simulink model "MBDMotorSystemUpd1MaxIaLmt"  (R2023a)
settings: Solver=VariableStepAuto  StartTime=0.0  StopTime=0.5  RelTol=1e-3
undefined symbols (not defined in the file or in its folder): CntFdqDcpMap, CntLdqDMap, CntTrqReqMap, DiscIntNeverNeededParam, Izc, Izr, MdlFluxMap, MdlTrqMap, Pos0
libraries: simulink x30, simulink_extras x6
(part 2 of 4)

== system MBDMotorSystemUpd1MaxIaLmt/PM Controller/IPM Trq To Id-Iq Request ==
  Vdc : Inport
  TrqIn : Inport  Port=2
  w : Inport  Port=3
  Time : Inport  Port=4
  Trigger : TriggerPort  VariantControl=Variant  PortDimensions=1
  Abs : Abs  SaturateOnIntegerOverflow=off
  Display : Display
  Gain : Gain  Gain=120/nP
  Gain1 : Gain  Gain=-1
  Id Map : Lookup_n-D  NumberOfTableDimensions=3  BreakpointsForDimension1=TrqIdx  BreakpointsForDimension2=NsIdx  BreakpointsForDimension3=VdcIdx  Table=IdMap  InternalRulePriority=Speed  RndMeth=Simplest
      settings: InputPortMap=u0,u1,u2
  Iq Map : Lookup_n-D  NumberOfTableDimensions=3  BreakpointsForDimension1=TrqIdx  BreakpointsForDimension2=NsIdx  BreakpointsForDimension3=VdcIdx  Table=IqMap  InternalRulePriority=Speed  RndMeth=Simplest
      settings: InputPortMap=u0,u1,u2
  Mux : Mux  Inputs=2
  Product : Product
  Product1 : Product
  Saturation Dynamic : simulink/Discontinuities/Saturation Dynamic  OutMin=[]  OutMax=[]  OutDataTypeStr=Inherit: Same as second input  OutDataType=fixdt(1, 16)  OutScaling=2^-10  DoSatur=off
  Sign : Signum
  Sign1 : Signum
  Torque Rate Limitter : Subsystem  mask{DltLmt=DltTrqLmt}
      mask prompts: DltLmt "変化率制限 [unit/s]"
  Trq Limt Map : Lookup_n-D  BreakpointsForDimension1=NsIdx  BreakpointsForDimension2=VdcIdx  BreakpointsForDimension3=VdcIdx  Table=MapLimitTrq  InternalRulePriority=Speed  RndMeth=Simplest
      settings: InputPortMap=u0,u1
  WtoF : Gain  Gain=1/(2*pi)
  TrqReq : Outport
  IdqReq : Outport  Port=2
  wires:
  Mux/1 -> IdqReq/1
  Id Map/1 -> Mux/1
  w/1 -> WtoF/1
  TrqIn/1 -> Torque Rate Limitter/1(In)
  Saturation Dynamic/1 -> Product/1, Id Map/1, Iq Map/1
  Gain1/1 -> Saturation Dynamic/3
  Vdc/1 -> [Vdc]
  [Vdc] -> Trq Limt Map/2
  [Nrpm] -> Iq Map/2, Id Map/2
  [Nrpm] -> Trq Limt Map/1
  Gain/1 -> Display/1, [Nrpm]
  [Vdc] -> Id Map/3, Iq Map/3
  Trq Limt Map/1 -> Gain1/1, Saturation Dynamic/1
  Torque Rate Limitter/1(Rate Limited) -> Abs/1, Sign1/1, Sign/1
  Time/1 -> Torque Rate Limitter/2(Time)
  Abs/1 -> Saturation Dynamic/2
  Product/1 -> TrqReq/1
  Sign/1 -> Product/2
  Product1/1 -> Mux/2
  Iq Map/1 -> Product1/1
  Sign1/1 -> Product1/2
  WtoF/1 -> Gain/1

== system MBDMotorSystemUpd1MaxIaLmt/PM Controller/LPF ==
  In : Inport  SampleTime=Ts
  Init : Inport  Port=2  SampleTime=Ts
  Constant : Constant  Value=Ts
  Constant1 : Constant  Value=tau
  Delay : Delay  DelayLength=1  InitialConditionSource=Input port
      settings: InputPortMap=u0,p4
  Divide1 : Product  Inputs=*/
  Divide3 : Product  Inputs=*/
  Product : Product
  Product1 : Product
  Sum1 : Sum
  Sum2 : Sum
  Sum3 : Sum  Inputs=-+
  Out : Outport
  wires:
  Constant1/1 -> Divide1/1, Sum1/2
  Constant/1 -> Sum1/1, Divide3/1
  Sum1/1 -> Divide1/2, Divide3/2
  Divide3/1 -> [kX]
  Divide1/1 -> [kY]
  In/1 -> Product/1
  [kX] -> Product/2
  Product/1 -> Sum3/1, Sum2/1
  Sum2/1 -> Out/1, Product1/1
  [kY] -> Product1/2
  Product1/1 -> Delay/1
  Delay/1 -> Sum2/2
  Init/1 -> Sum3/2
  Sum3/1 -> Delay/2

== system MBDMotorSystemUpd1MaxIaLmt/PM Controller/Modulator ==
  Vdc : Inport
  Vdq* : Inport  Port=2
  Th [deg.] : Inport  Port=3
  w : Inport  Port=4
  Tc : Inport  Port=5
  Trigger : TriggerPort  TriggerType=falling  VariantControl=Variant
  DQ to UVW : Subsystem
  Divide : Product  Inputs=*/
  Gain : Gain  Gain=0.5
  Gain2 : Gain  Gain=1.5
  IsOvrMod : Constant  Value=0
  Over Modulation : Subsystem
  Product : Product
  Saturation : Saturate  UpperLimit=inf  LowerLimit=1  LinearizeAsGain=off
  Sum : Sum  Inputs=|++
  Sum7 : Sum  Inputs=|+-
  TypePWM : Constant  Value=0
  Vz Correction : Subsystem
  Muvw : Outport
  Vuvw* : Outport  Port=2
  wires:
  Gain/1 -> Vz Correction/3(MaxVa), Divide/2
  Sum/1 -> Divide/1
  Vz Correction/1(Vz) -> Sum/2
  DQ to UVW/1(UVW) -> Sum/1, Vuvw*/1, Vz Correction/2(VaReq)
  Vdq*/1 -> DQ to UVW/1(dq)
  Vdc/1 -> Saturation/1
  Saturation/1 -> Gain/1
  Product/1 -> Gain2/1
  Th [deg.]/1 -> Sum7/1
  Sum7/1 -> DQ to UVW/2(Th)
  w/1 -> Product/1
  Tc/1 -> Product/2
  Gain2/1 -> Sum7/2
  Divide/1 -> Over Modulation/3(Mr)
  IsOvrMod/1 -> Over Modulation/1(Is OvrMod)
  TypePWM/1 -> Over Modulation/2(PWM Mode), Vz Correction/1(PWM Mode)
  Over Modulation/1(Mr*) -> Muvw/1

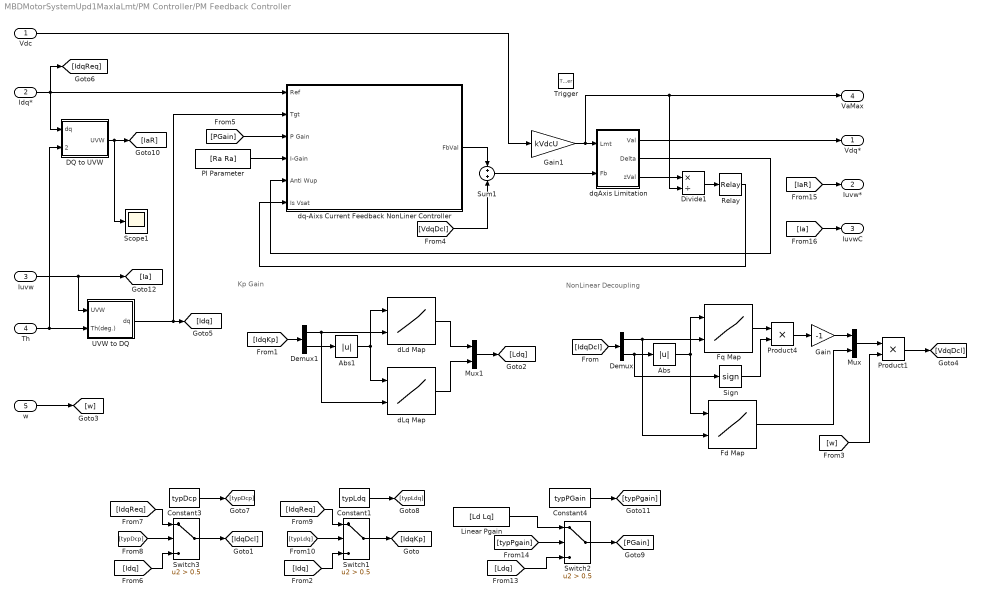
== system MBDMotorSystemUpd1MaxIaLmt/PM Controller/PM Feedback Controller ==
  note: Kp Gain
  note: NonLinear Decoupling
  Vdc : Inport
  Idq* : Inport  Port=2
  Iuvw : Inport  Port=3
  Th : Inport  Port=4
  w : Inport  Port=5
  Trigger : TriggerPort  TriggerType=falling  VariantControl=Variant  PortDimensions=1
  Abs : Abs  SaturateOnIntegerOverflow=off
  Abs1 : Abs  SaturateOnIntegerOverflow=off
  Constant1 : Constant  Value=typLdq
  Constant3 : Constant  Value=typDcp
  Constant4 : Constant  Value=typPGain
  DQ to UVW : Subsystem
  Demux : Demux  Outputs=2
  Demux1 : Demux  Outputs=2
  Divide1 : Product  Inputs=*/
  Fd Map : Lookup_n-D  BreakpointsForDimension1=axIqY  BreakpointsForDimension2=axIdX  Table=mIdqToFd  InternalRulePriority=Speed  RndMeth=Simplest
      settings: InputPortMap=u0,u1
  Fq Map : Lookup_n-D  BreakpointsForDimension1=axIqY  BreakpointsForDimension2=axIdX  Table=mIdqToFq  InternalRulePriority=Speed  RndMeth=Simplest
      settings: InputPortMap=u0,u1
  Gain : Gain  Gain=-1
  Gain1 : Gain  Gain=kVdcU
  Linear Pgain : Constant  Value=[Ld Lq]
  Mux : Mux  Inputs=2
  Mux1 : Mux  Inputs=2
  PI Parameter : Constant  Value=[Ra Ra]
  Product1 : Product
  Product4 : Product
  Relay : Relay  OnSwitchValue=0.98  OffSwitchValue=0.95
  Scope1 : Scope
  Sign : Signum
  Sum1 : Sum  Inputs=+|+
  Switch1 : Switch  Criteria=u2 > Threshold  Threshold=0.5  SaturateOnIntegerOverflow=off  InputSameDT=off
  Switch2 : Switch  Criteria=u2 > Threshold  Threshold=0.5  SaturateOnIntegerOverflow=off  InputSameDT=off
  Switch3 : Switch  Criteria=u2 > Threshold  Threshold=0.5  SaturateOnIntegerOverflow=off  InputSameDT=off
  UVW to DQ : Subsystem
  dLd Map : Lookup_n-D  BreakpointsForDimension1=axIdXdL  BreakpointsForDimension2=axIqYdL  Table=mIdqToLd  InternalRulePriority=Speed  RndMeth=Simplest
      settings: InputPortMap=u0,u1
  dLq Map : Lookup_n-D  BreakpointsForDimension1=axIdXdL  BreakpointsForDimension2=axIqYdL  Table=mIdqToLq  InternalRulePriority=Speed  RndMeth=Simplest
      settings: InputPortMap=u0,u1
  dq-Aixs Current Feedback NonLiner Controller : Subsystem  mask{KcDt=KcDt, KcQt=KcQt, KcDw=KcDw, KcQw=KcQw}
      mask prompts: KcDt "Id Cut off Gain [rad./s]"; KcQt "Iq Cut off Gain [rad./s]"; KcDw "Id Cut off Gain [rad./s]"; KcQw "Iq Cut off Gain [rad./s]"
      mask init:
      | KcT=[KcDt KcQt];
      |     KcW=[KcDw KcQw];
      mask DialogControl Container1 Prompt: Current Feedback Gain
      mask DialogControl Container2 Prompt: MTPA
      mask DialogControl Container3 Prompt: Field Weakening
      mask Display:
      | disp(['dq-Axis Current Feedback\nControler\n\n', ...
      |       sprintf('MTPA - d:%g / q:%g [rad./s]\n',KcDt,KcQt), ...
      |       sprintf('FdWk - d:%g / q:%g [rad./s]\n',KcDw,KcQw), ...
      |       '']);
  dqAxis Limitation : Subsystem
  Vdq* : Outport
  Iuvw* : Outport  Port=2
  IuvwC : Outport  Port=3
  VaMax : Outport  Port=4
  wires:
  DQ to UVW/1(UVW) -> [IaR], Scope1/1
  Th/1 -> DQ to UVW/2(Th. [deg.]), UVW to DQ/2(Th(deg.))
  Iuvw/1 -> [Ia], UVW to DQ/1(UVW)
  Gain1/1 -> Divide1/2, VaMax/1, dqAxis Limitation/1(Lmt)
  Sum1/1 -> dqAxis Limitation/2(Fb)
  dqAxis Limitation/1(Val) -> Vdq*/1
  Idq*/1 -> [IdqReq], DQ to UVW/1(dq), dq-Aixs Current Feedback NonLiner Controller/1(Ref)
  Vdc/1 -> Gain1/1
  dqAxis Limitation/2(Delta) -> dq-Aixs Current Feedback NonLiner Controller/5(Anti Wup)
  UVW to DQ/1(dq) -> [Idq], dq-Aixs Current Feedback NonLiner Controller/2(Tgt)
  Gain/1 -> Mux/1
  Fd Map/1 -> Mux/2
  dLd Map/1 -> Mux1/1
  dLq Map/1 -> Mux1/2
  [IdqDcl] -> Demux/1
  [IdqKp] -> Demux1/1
  Mux1/1 -> [Ldq]
  w/1 -> [w]
  [w] -> Product1/2
  [VdqDcl] -> Sum1/2
  Switch3/1 -> [IdqDcl]
  [Idq] -> Switch3/3
  [IdqReq] -> Switch3/1
  [typDcp] -> Switch3/2
  Constant3/1 -> [typDcp]
  [typLdq] -> Switch1/2
  [Idq] -> Switch1/3
  [IdqReq] -> Switch1/1
  Switch1/1 -> [IdqKp]
  Constant1/1 -> [typLdq]
  [Ldq] -> Switch2/3
  Linear Pgain/1 -> Switch2/1
  Switch2/1 -> [PGain]
  Constant4/1 -> [typPgain]
  [typPgain] -> Switch2/2
  [PGain] -> dq-Aixs Current Feedback NonLiner Controller/3(P Gain)
  PI Parameter/1 -> dq-Aixs Current Feedback NonLiner Controller/4(I-Gain)
  Divide1/1 -> Relay/1
  dqAxis Limitation/3(zVal) -> Divide1/1
  Relay/1 -> dq-Aixs Current Feedback NonLiner Controller/6(Is Vsat)
  Demux/1 -> Fd Map/2, Fq Map/2
  Demux/2 -> Sign/1, Abs/1
  Product4/1 -> Gain/1
  Fq Map/1 -> Product4/1
  Sign/1 -> Product4/2
  Abs/1 -> Fd Map/1, Fq Map/1
  Demux1/2 -> Abs1/1
  Abs1/1 -> dLq Map/1, dLd Map/1
  Demux1/1 -> dLd Map/2, dLq Map/2
  Product1/1 -> [VdqDcl]
  Mux/1 -> Product1/1
  dq-Aixs Current Feedback NonLiner Controller/1(FbVal) -> Sum1/1
  [IaR] -> Iuvw*/1
  [Ia] -> IuvwC/1

== system MBDMotorSystemUpd1MaxIaLmt/PM Controller/PWM Timer ==
  Req : Inport  PortDimensions=3
  Fc : Inport  Port=2
  Iuvw : Inport  Port=3
  Base Modulator : Subsystem  mask{lTypTrigger=1: 山}
      mask prompts: lTypTrigger "更新トリガ"
      mask TypeOptions lTypTrigger: sampler/lTypTrigger
  Dead  Time : Constant  Value=[Td; -Td]
  DeadTime Correction : Subsystem  mask{IsDeadTimeCorrection=on, vThr=vThr}
      mask prompts: IsDeadTimeCorrection "DeadTime補償有効"; vThr "補償方向電流閾値"
      mask init:
      | if strcmp(get_param(gcbh,'IsDeadTimeCorrection'),'on')
      |     kCrctTd=1;
      | else
      |     kCrctTd=0;
      | end
  Demux : Demux  Outputs=2
  Demux1 : Demux  Outputs=3
  Demux2 : Demux  Outputs=3
  Gain : Gain  Gain=2
  Mux{1..4} (4 alike) : Mux  Inputs=2
  Mux5 : Mux  Inputs=3
  PWM Sampler : Subsystem  TreatAsAtomicUnit=on
  PWM Status : Scope  NumInputPorts=4
  Product1 : Product
  Relational Operator : RelationalOperator  OutDataTypeStr=boolean  RndMeth=Simplest  InputSameDT=off
  Relational Operator1 : RelationalOperator  Operator=<=  OutDataTypeStr=boolean  RndMeth=Simplest  InputSameDT=off
  Signal Offset : Subsystem
  Sum1 : Sum  Inputs=|++
  Sum2 : Sum  Inputs=|++
  Trg : Outport
  PWM : Outport  Port=2
  Tc : Outport  Port=3
  wires:
  [Trg] -> PWM Status/3
  [ModV] -> PWM Status/2
  Mux4/1 -> [ModV]
  [CrcTd] -> PWM Status/4
  Sum2/1 -> Mux4/2, Relational Operator/1, Relational Operator1/1
  PWM Sampler/1(s) -> Sum2/1
  DeadTime Correction/1(Tdc) -> Sum2/2, [CrcTd]
  Iuvw/1 -> DeadTime Correction/2(Iuvw)
  Base Modulator/1("Trigger ") -> [Trg], PWM Sampler/Trigger, Trg/1
  Sum1/1 -> Mux4/1, Demux/1
  Product1/1 -> Sum1/2, DeadTime Correction/1(Tdcs)
  Base Modulator/2(Carrier) -> Sum1/1
  Fc/1 -> Product1/1, Base Modulator/1(Fc)
  Gain/1 -> Product1/2
  Dead  Time/1 -> Gain/1
  Mux5/1 -> Signal Offset/1(puvw), PWM/1
  Req/1 -> PWM Sampler/1(v)
  Mux3/1 -> Mux5/3  "Pw"
  Mux2/1 -> Mux5/2  "Pv"
  Mux1/1 -> Mux5/1  "Pu"
  Signal Offset/1(Pwm SigOuts) -> PWM Status/1
  Demux2/3 -> Mux3/2
  Demux2/2 -> Mux2/2
  Demux2/1 -> Mux1/2
  Demux1/3 -> Mux3/1
  Demux1/2 -> Mux2/1
  Demux1/1 -> Mux1/1
  Relational Operator1/1 -> Demux2/1
  Demux/2 -> Relational Operator1/2
  Demux/1 -> Relational Operator/2
  Relational Operator/1 -> Demux1/1
  Base Modulator/3(Tc) -> Tc/1

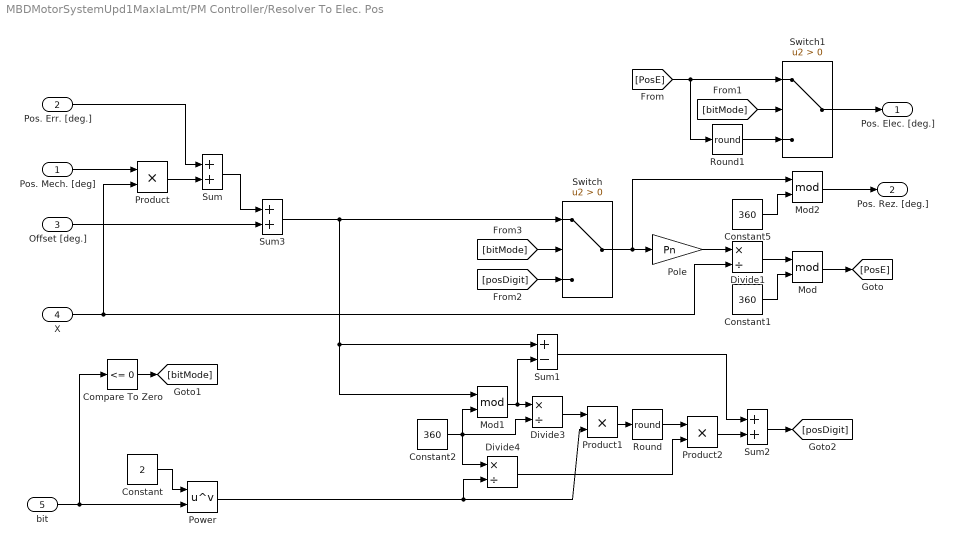
== system MBDMotorSystemUpd1MaxIaLmt/PM Controller/Resolver To Elec. Pos ==
  Pos. Mech. [deg] : Inport
  Pos. Err. [deg.] : Inport  Port=2
  Offset [deg.] : Inport  Port=3
  X : Inport  Port=4
  bit : Inport  Port=5
  Compare To Zero : simulink/Logic and Bit Operations/Compare To Zero  relop=<=  OutDataTypeStr=uint8
  Constant : Constant  Value=2
  Constant1 : Constant  Value=360
  Constant2 : Constant  Value=360
  Constant5 : Constant  Value=360
  Divide1 : Product  Inputs=*/
  Divide3 : Product  Inputs=*/
  Divide4 : Product  Inputs=*/
  Mod : Math  Operator=mod
  Mod1 : Math  Operator=mod
  Mod2 : Math  Operator=mod
  Pole : Gain  Gain=Pn
  Power : Math  Operator=pow
  Product : Product
  Product1 : Product
  Product2 : Product
  Round : Rounding  Operator=round
  Round1 : Rounding  Operator=round
  Sum : Sum
  Sum1 : Sum  Inputs=+-
  Sum2 : Sum
  Sum3 : Sum
  Switch : Switch  Criteria=u2 > Threshold  SaturateOnIntegerOverflow=off  InputSameDT=off
  Switch1 : Switch  Criteria=u2 > Threshold  SaturateOnIntegerOverflow=off  InputSameDT=off
  Pos. Elec. [deg.] : Outport
  Pos. Rez. [deg.] : Outport  Port=2
  wires:
  Pos. Mech. [deg]/1 -> Product/1
  Power/1 -> Divide4/2, Product1/2
  X/1 -> Product/2, Divide1/2
  bit/1 -> Power/2, Compare To Zero/1
  Constant/1 -> Power/1
  Constant1/1 -> Mod/2
  Product/1 -> Sum/2
  Switch/1 -> Mod2/1, Pole/1
  Pole/1 -> Divide1/1
  Divide1/1 -> Mod/1
  Round1/1 -> Switch1/3
  Switch1/1 -> Pos. Elec. [deg.]/1
  Mod/1 -> [PosE]
  [PosE] -> Round1/1, Switch1/1
  [bitMode] -> Switch1/2
  [posDigit] -> Switch/3
  Constant2/1 -> Divide4/1, Divide3/2, Mod1/2
  Compare To Zero/1 -> [bitMode]
  [bitMode] -> Switch/2
  Mod2/1 -> Pos. Rez. [deg.]/1
  Constant5/1 -> Mod2/2
  Pos. Err. [deg.]/1 -> Sum/1
  Mod1/1 -> Sum1/2, Divide3/1
  Divide3/1 -> Product1/1
  Product1/1 -> Round/1
  Round/1 -> Product2/1
  Divide4/1 -> Product2/2
  Product2/1 -> Sum2/2
  Sum1/1 -> Sum2/1
  Sum2/1 -> [posDigit]
  Sum3/1 -> Mod1/1, Sum1/1, Switch/1
  Offset [deg.]/1 -> Sum3/2
  Sum/1 -> Sum3/1

== system MBDMotorSystemUpd1MaxIaLmt/PM Controller/Resolver Settings ==
  Pos. Mech. [deg.] : Inport
  Bit : Constant  Value=10
  Bus Creator : BusCreator  Inputs=3
  Constant : Constant  Value=0
  Constant1 : Constant  Value=0
  Constant4 : Constant  Value=360
  Err Stt : Constant
  Fail : Step  Time=1.2  SampleTime=0
  Fail Speed a [rpm] : Constant  Value=0
  Fail Speed b [rpm] : Constant  Value=30
  Fail Stt : Constant
  Manual Switch{,1..3} (4 alike) : ManualSwitch
  Mod1 : Math  Operator=mod
  Offset : Constant  Value=0
  Product : Product
  Resolver Error : Subsystem
  Resolver Fail : Subsystem
  X : Constant  Value=50
  Pos. Mech. [deg] : Outport
  Err. [deg.] : Outport  Port=2
  Ia Sensor Parm. : Outport  Port=3
  wires:
  Bus Creator/1 -> Ia Sensor Parm./1
  Pos. Mech. [deg.]/1 -> Product/2, Resolver Fail/1(Pos. Mech. [deg.])
  Resolver Error/1(Err. [deg.]) -> Err. [deg.]/1
  Offset/1 -> Bus Creator/1  "Offset"
  X/1 -> [x], Bus Creator/2  "X"
  Bit/1 -> Bus Creator/3  "Bit"
  Resolver Fail/1(Pos. Mech. [deg]) -> Pos. Mech. [deg]/1
  Fail Speed a [rpm]/1 -> Manual Switch/1
  Fail Speed b [rpm]/1 -> Manual Switch/2
  Manual Switch/1 -> Resolver Fail/2(Fail Speed [rpm])
  Fail Stt/1 -> Manual Switch1/1
  Fail/1 -> Manual Switch1/2
  Manual Switch2/1 -> Resolver Fail/3(Fail)
  Constant/1 -> Manual Switch2/1
  Manual Switch1/1 -> Manual Switch2/2
  Constant1/1 -> Manual Switch3/1
  Err Stt/1 -> Manual Switch3/2
  Manual Switch3/1 -> Resolver Error/2(Fail)
  [x] -> Product/1
  Constant4/1 -> Mod1/2
  Product/1 -> Mod1/1
  Mod1/1 -> Resolver Error/1(Pos Rez. [deg.])

== system MBDMotorSystemUpd1MaxIaLmt/PM Controller/TrgPos ==
  Pos (deg.) : Inport
  Trigger : TriggerPort  TriggerType=falling  VariantControl=Variant
  Pos (Smpled) : Outport
  wires:
  Pos (deg.)/1 -> Pos (Smpled)/1

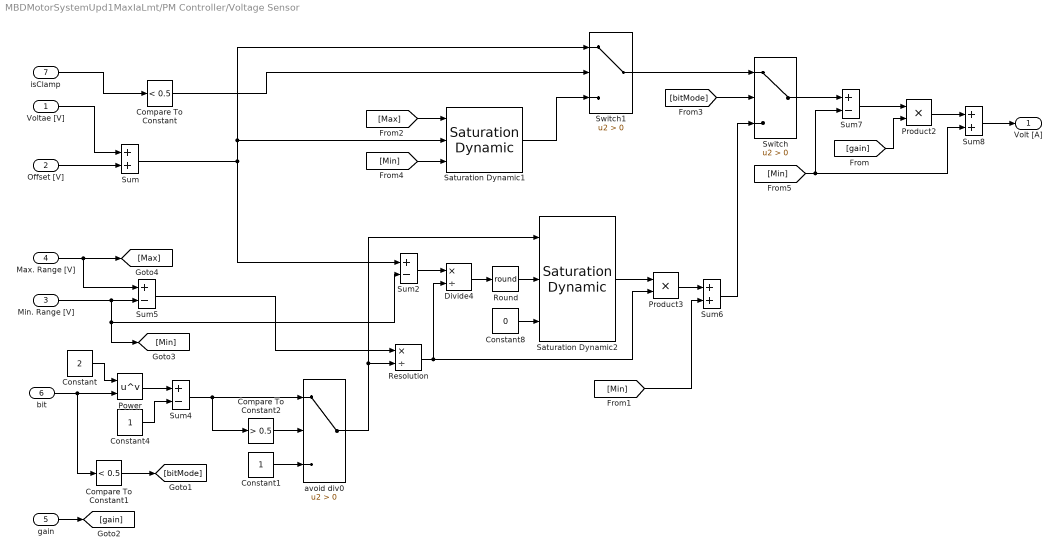
== system MBDMotorSystemUpd1MaxIaLmt/PM Controller/Voltage Sensor ==
  Voltae [V] : Inport
  Offset [V] : Inport  Port=2
  Min. Range [V] : Inport  Port=3
  Max. Range [V] : Inport  Port=4
  gain : Inport  Port=5
  bit : Inport  Port=6
  isClamp : Inport  Port=7
  Compare To Constant : simulink/Logic and Bit Operations/Compare To Constant  relop=<  const=0.5  OutDataTypeStr=boolean
  Compare To Constant1 : simulink/Logic and Bit Operations/Compare To Constant  relop=<  const=0.5  OutDataTypeStr=boolean
  Compare To Constant2 : simulink/Logic and Bit Operations/Compare To Constant  relop=>  const=0.5  OutDataTypeStr=boolean
  Constant : Constant  Value=2
  Constant1 : Constant
  Constant4 : Constant
  Constant8 : Constant  Value=0
  Divide4 : Product  Inputs=*/
  Power : Math  Operator=pow
  Product2 : Product
  Product3 : Product
  Resolution : Product  Inputs=*/
  Round : Rounding  Operator=round
  Saturation Dynamic1 : simulink/Discontinuities/Saturation Dynamic  OutMin=[]  OutMax=[]  OutDataTypeStr=Inherit: Same as second input  OutDataType=fixdt(1, 16)  OutScaling=2^-10  DoSatur=off
  Saturation Dynamic2 : simulink/Discontinuities/Saturation Dynamic  OutMin=[]  OutMax=[]  OutDataTypeStr=Inherit: Same as second input  OutDataType=fixdt(1, 16)  OutScaling=2^-10  DoSatur=off
  Sum : Sum
  Sum{2,4..5,7} (4 alike) : Sum  Inputs=+-
  Sum6 : Sum
  Sum8 : Sum
  Switch : Switch  Criteria=u2 > Threshold  SaturateOnIntegerOverflow=off  InputSameDT=off
  Switch1 : Switch  Criteria=u2 > Threshold  SaturateOnIntegerOverflow=off  InputSameDT=off
  "avoid div0  " : Switch  Criteria=u2 > Threshold  SaturateOnIntegerOverflow=off  InputSameDT=off
  Volt [A] : Outport
  wires:
  Constant/1 -> Power/1
  Compare To Constant1/1 -> [bitMode]
  [bitMode] -> Switch/2
  Offset [V]/1 -> Sum/2
  Voltae [V]/1 -> Sum/1
  Power/1 -> Sum4/1
  Constant4/1 -> Sum4/2
  Divide4/1 -> Round/1
  isClamp/1 -> Compare To Constant/1
  Switch1/1 -> Switch/1
  Compare To Constant/1 -> Switch1/2
  gain/1 -> [gain]
  Switch/1 -> Sum7/1
  [gain] -> Product2/2
  Min. Range [V]/1 -> [Min], Sum2/2, Sum5/2
  bit/1 -> Compare To Constant1/1, Power/2
  Max. Range [V]/1 -> [Max], Sum5/1
  Sum5/1 -> Resolution/1
  Sum/1 -> Switch1/1, Saturation Dynamic1/2, Sum2/1
  Sum2/1 -> Divide4/1
  Resolution/1 -> Product3/2, Divide4/2
  Round/1 -> Saturation Dynamic2/2
  Constant8/1 -> Saturation Dynamic2/3
  Saturation Dynamic2/1 -> Product3/1
  Product3/1 -> Sum6/1
  [Min] -> Sum6/2
  [Max] -> Saturation Dynamic1/1
  [Min] -> Saturation Dynamic1/3
  Saturation Dynamic1/1 -> Switch1/3
  Sum6/1 -> Switch/3
  [Min] -> Sum8/2, Sum7/2
  Product2/1 -> Sum8/1
  Sum8/1 -> Volt [A]/1
  Sum7/1 -> Product2/1
  Compare To Constant2/1 -> "avoid div0  "/2
  Constant1/1 -> "avoid div0  "/3
  Sum4/1 -> Compare To Constant2/1, "avoid div0  "/1
  "avoid div0  "/1 -> Saturation Dynamic2/1, Resolution/2

== system MBDMotorSystemUpd1MaxIaLmt/PM Controller/Voltage Settings  ==
  Bit : Constant  Value=12
  Bus Creator : BusCreator  Inputs=6
  Error Gain : Constant  Value=0.8
  Gain : Constant
  IsClamp : Constant
  Manual Switch : ManualSwitch
  Max. Range : Constant  Value=1000
  Min. Range : Constant  Value=0
  Offset : Constant  Value=0
  Ia Sensor Parm. : Outport
  wires:
  Offset/1 -> Bus Creator/1  "Offset"
  Bus Creator/1 -> Ia Sensor Parm./1
  Min. Range/1 -> Bus Creator/2  "Min"
  Gain/1 -> Manual Switch/1  "Gain"
  Manual Switch/1 -> [gain]
  Error Gain/1 -> Manual Switch/2
  Max. Range/1 -> Bus Creator/3  "Max"
  [gain] -> Bus Creator/4  "Gain"
  Bit/1 -> Bus Creator/5  "Bit"
  IsClamp/1 -> Bus Creator/6  "IsClamp"

== system MBDMotorSystemUpd1MaxIaLmt/Power Source/Power Source Cable Cs ==
  note: コンデンサオープン時モデル
  note: 正常時モデル
  Vb0 : Inport
  I Load : Inport  Port=2
  fail : Inport  Port=3
  Bus Creator : BusCreator  Inputs=5
  Bus Selector : BusSelector  OutputSignals=Vdc
  Bus Selector1 : BusSelector  OutputSignals=Ib
  Cable LR : Subsystem  mask{LcN=LcN, IsSetRC=Off, RcM=RcM}
      mask prompts: LcN "インダクタンス [nH]"; IsSetRC "Rc考慮"; RcM "抵抗 [mΩ]"
      mask init:
      | % disp('>>>>>>>> LR Cable Initialized. Start')
      |     % fprintf('CS: %8.f [uF], ESR:%8.f [mΩ], IR:%8.f [MΩ]\n',CsU, ESRm, IRM)
      |     hb = getSimulinkBlockHandle([gcb, '/vLc']);
      |     set_param(hb, "Value", num2str(LcN * 1.0e-9));
      |     hb = getSimulinkBlockHandle([gcb, '/vRc']);
      |     set_param(hb, "Value", num2str(RcM * 1.0e-3));
      | 
      |     % x = get_param(gcbh,"RcUse");
      |     % if strcmpi(x, "On")
      |     %     V = Simulink.Parameter(1)
      |     % else
      |     %     V = Simulink.Parameter(2)
      |     % end
      |     % disp('>>>>>>>> LR Cable Initialized. End')
      mask Callback LcN:
      | % disp('>>>>>>>> LcN Callback Start.')
      |     hb = getSimulinkBlockHandle([gcb, '/vLc']);
      |     LcN = str2double(get_param(gcbh, "LcN"));
      |     % get_param(hb, "Name")
      |     set_param(hb, "Value", num2str(LcN * 1.0e-9));
      |     % disp('>>>>>>>> LcN Callback End.')
      mask TypeOptions IsSetRC: Off | On
      mask Callback IsSetRC:
      | % disp('>>>>>>>> RcUse Callback Start.')
      |     stt = get_param(gcbh, "IsSetRC");
      |     hb = getSimulinkBlockHandle([gcb, '/IsRc']);
      |     set_param(hb, 'LabelModeActiveChoice', stt)
      |     % set_param(bdroot, 'SimulationCommand', 'update')
      |     % disp('>>>>>>>> RcUse Callback End.')
      mask Callback RcM:
      | hb = getSimulinkBlockHandle([gcb, '/vRc']);
      |     RcM = str2double(get_param(gcbh, "RcM"));
      |     set_param(hb, "Value", num2str(RcM * 1.0e-3));
      mask DialogControl ParameterGroupVar Prompt: パラメーター
      mask Display:
      | ss = sprintf('Cable LR');
      | % tn = [gcb, '/IsRc'];
      | % hn = getSimulinkBlockHandle(tn);
      | % stt = get_param(hn, "LabelModeActiveChoice");
      | stt = get_param(gcbh, "IsSetRC");
      | if strcmpi(stt, 'On')
      |     ss = sprintf('%s\nRL', ss);
      | else
      |     ss = sprintf('%s\nL', ss);
      | end
      | 
      | ss = sprintf('%s\n %s[nH]', ss, ...
      |         get_param(gcbh, "LcN"));
      | if strcmpi(stt, 'On')
      |     ss = sprintf('%s\n%s[mΩ]', ss,get_param(gcbh,"RcM"));
      | end
      | disp(ss)
  Cable LRC : Subsystem  mask{LcN=LcNo, CcN=CcNo, IsSetRc=Off, RcM=RcMo}
      mask prompts: LcN "配線インダクタンス [nH]"; CcN "配線容量 [nF]"; IsSetRc "Rc考慮"; RcM "抵抗 [mΩ]"
      mask init:
      | hb = getSimulinkBlockHandle([gcb, '/vLc']);
      |     set_param(hb, "Value", num2str(LcN * 1.0e-9));
      |     hb = getSimulinkBlockHandle([gcb, '/vRc']);
      |     set_param(hb, "Value", num2str(RcM * 1.0e-3));
      |     hb = getSimulinkBlockHandle([gcb, '/vCc']);
      |     set_param(hb, "Value", num2str(CcN * 1.0e-9));
      mask Callback LcN:
      | hb = getSimulinkBlockHandle([gcb, '/vLc']);
      |     LcN = str2double(get_param(gcbh, "LcN"));
      |     set_param(hb, "Value", num2str(LcN * 1.0e-9));
      mask Callback CcN:
      | hb = getSimulinkBlockHandle([gcb, '/vCc']);
      |     CcN = str2double(get_param(gcbh, "CcN"));
      |     set_param(hb, "Value", num2str(CcN * 1.0e-9));
      mask TypeOptions IsSetRc: Off | On
      mask Callback IsSetRc:
      | stt = get_param(gcbh, "IsSetRc");
      |     hb = getSimulinkBlockHandle([gcb, '/IsRc']);
      |     set_param(hb, 'LabelModeActiveChoice', stt)
      mask Callback RcM:
      | hb = getSimulinkBlockHandle([gcb, '/vRc']);
      |     RcM = str2double(get_param(gcbh, "RcM"));
      |     set_param(hb, "Value", num2str(RcM * 1.0e-3));
      mask DialogControl ParameterGroupVar Prompt: パラメーター
      mask Display:
      | tn = [gcb, '/IsRc'];
      | hn = getSimulinkBlockHandle(tn);
      | stt = get_param(hn, "LabelModeActiveChoice");
      | if strcmpi(stt, 'On')
      |     ss = sprintf('Cable Vout.\nRLC');
      | else
      |     ss = sprintf('Cable LRC.\nLC');
      | end
      | 
      | ss = sprintf('%s\n %s[nH] / %s[nF]', ss, ...
      |         get_param(gcbh, "LcN"), get_param(gcbh, "CcN"));
      | if strcmpi(stt, 'On')
      |     ss = sprintf('%s\n%s[mΩ]', ss,get_param(gcbh,"RcM"));
      | end
      | disp(ss)
  Compare To Constant1 : simulink/Logic and Bit Operations/Compare To Constant  relop=<  const=0.5  OutDataTypeStr=boolean
  Constant : Constant  Value=0
  Cs No ESL : Subsystem  mask{CsU=CsU, IsEnableESR=Off, ESRm=ESRm, IsEnableIR=Off, IRM=IRM}
      mask prompts: CsU "コンデンサ容量 [uF]"; IsEnableESR "ESR考慮"; ESRm "ESR [mΩ]"; IsEnableIR "IR考慮"; IRM "IR [MΩ]"
      mask init:
      | Cs  = CsU  * 1.0e-6;
      |     ESR = ESRm * 1.0e-3;
      |     IR  = IRM  * 1.0e6;
      mask TypeOptions IsEnableESR: IsESR/LabelModeActiveChoice | IsESRini/LabelModeActiveChoice
      mask TypeOptions IsEnableIR: isIR/LabelModeActiveChoice
      mask DialogControl ParameterGroupVar Prompt: パラメーター
      mask Display:
      | ss = 'Cs No ESL.';
      | if strcmpi(get_param(gcbh, "IsEnableESR"), 'On')
      |     ss = sprintf('%s\nESR', ss);
      | end
      | if strcmpi(get_param(gcbh, "IsEnableIR"), 'On')
      |     if contains(ss, 'ESR', 'IgnoreCase',true)
      |         ss = sprintf('%s / IR', ss);
      |     else
      |         ss = sprintf('%s\nIR', ss);
      |     end
      | end
      | % cv = evalin("caller","Cs")*1e6;
      | % ss =sprintf('%s\n %g[uF]', ss, cv);
      | ss =sprintf('%s\n %s[uF]', ss, get_param(gcbh, "CsU"));
      | 
      | if strcmpi(get_param(gcbh, "IsEnableESR"), 'On')
      |     % rv = evalin("caller","ESR")*1e3;
      |     % ss = sprintf('%s\n%g[mΩ]', ss, rv);
      |     ss =sprintf('%s\n %s[mΩ]', ss, get_param(gcbh, "ESRm"));
      | end
      | if strcmpi(get_param(gcbh, "IsEnableIR"), 'On')
      |     if contains(ss, 'ESR', 'IgnoreCase',true)
      |         ss = sprintf('%s / ', ss);
      |     else
      |         ss = sprintf('%s\n', ss);
      |     end
      |     % rv = evalin("caller","IR")*1e-6;
      |     % ss = sprintf('%s%g[MΩ]', ss, rv);
      |     ss = sprintf('%s%s[MΩ]', ss, get_param(gcbh, "IRM"));
      | end
      | 
      | disp(ss)
      | % if strcmpi(get_param(gcbh, "IsEnableESR"), 'On')
      | %     ss = sprintf('%s\nESR', ss);
      | % end
      | % if strcmpi(get_param(gcbh, "IsEnableIR"), 'On')
      | %     if contains(ss, 'ESR', 'IgnoreCase',true)
      | %         ss = sprintf('%s / IR', ss);
      | %     else
      | %         ss = sprintf('%s\nIR', ss);
      | %     end
      | % end
  Demux : Demux  Outputs=2
  Eb Vout : Subsystem  mask{TypeSource=PS, Cb=Cb, Rb=Rb, IsZinM=Off, Cm=Cm, Rm=Rm, IsZinD=Off, Cd=Cd, Rd=Rd}
      mask prompts: TypeSource "電源ソース"; Cb "キャパシタ容量 [F]"; Rb "内部抵抗 [Ω]"; IsZinM "電荷移動特性考慮"; Cm "容量 [F]"; Rm "抵抗 [Ω]"; IsZinD "拡散特性考慮"; Cd "容量 [F]"; Rd "抵抗 [Ω]"
      mask TypeOptions TypeSource: Source/LabelModeActiveChoice
      mask TypeOptions IsZinM: Zcm/LabelModeActiveChoice
      mask TypeOptions Cm: Zm/Cz
      mask TypeOptions Rm: Zm/Rz
      mask TypeOptions IsZinD: Zcd/LabelModeActiveChoice
      mask TypeOptions Cd: Zd/Cz
      mask TypeOptions Rd: Zd/Rz
      mask DialogControl ParameterGroupVar Prompt: パラメーター
      mask DialogControl Container3 Prompt: 内部インピーダンス
      mask DialogControl Container4 Prompt: 電荷移動特性
      mask DialogControl Container5 Prompt: 拡散特性
      mask Display:
      | ss = get_param(gcbh, "TypeSource");
      | stm = get_param(gcbh, "IsZinM");
      | if strcmpi(stm, 'On')
      |     ss = sprintf('%s\n Zm', ss);
      | end
      | std = get_param(gcbh, "IsZinD");
      | if strcmpi(std, 'On')
      |     if strcmpi(stm, 'On')
      |         ss = sprintf('%s / Zd', ss);
      |     else
      |         ss = sprintf('%s\n Zd', ss);
      |     end
      | end
      | ss = sprintf('%s\n %s[Ω]', ss, get_param(gcbh, "Rb"));
      | if strcmpi(stm, 'On')
      |     ss = sprintf('%s\n %s[F] / %s[Ω]', ss, ...
      |         get_param(gcbh, "Cm"), get_param(gcbh, "Rm"));
      | end
      | if strcmpi(std, 'On')
      |     ss = sprintf('%s\n %s[F] / %s[Ω]', ss, ...
      |         get_param(gcbh, "Cd"), get_param(gcbh, "Rd"));
      | end
      | fprintf('Batt. Vout\n%s', ss)
  Mux : Mux  Inputs=2
  Mux1 : Mux  Inputs=2
  Switch : Switch  Criteria=u2 > Threshold  SaturateOnIntegerOverflow=off  InputSameDT=off
  Switch1 : Switch  Criteria=u2 > Threshold  SaturateOnIntegerOverflow=off  InputSameDT=off
  Vdc : Outport
  Ib : Outport  Port=2
  Stt : Outport  Port=3
  wires:
  Eb Vout/1(Vb) -> Cable LRC/1(Vin), Cable LR/1(Vin)
  Demux/2 -> Bus Creator/2  "Ib"
  Eb Vout/2(Stt) -> [SttPSV]
  Cs No ESL/1(Vdc) -> Cable LR/2(Vo), Cable LRC/3(V0), Mux/1  "Vdc"
  Cable LR/1(Ib) -> Cs No ESL/2(Ib), Mux/2  "Ib"
  I Load/1 -> Cs No ESL/1(I Load), Cable LRC/2(Io)
  Vb0/1 -> Eb Vout/1(Vb0), Cs No ESL/3(V0in)
  Cs No ESL/2(Stt) -> [SttCsV]
  Bus Selector/1 -> Vdc/1  "<Vdc>"
  Bus Creator/1 -> Bus Selector/1, Bus Selector1/1, Stt/1  "PsStt"
  [Ib] -> Eb Vout/2(Ib)
  Cable LRC/1(Vo) -> Mux1/1  "Vdc"
  Cable LRC/2(Ib) -> Mux1/2  "Ib"
  Cable LRC/3(Stt) -> [SttCBL1]
  Demux/1 -> Bus Creator/1  "Vdc"
  [SttPSV] -> Bus Creator/4
  [SttCsV] -> Bus Creator/3
  Mux1/1 -> Switch/3
  Switch1/1 -> Bus Creator/5
  Cable LR/2(Stt) -> [SttCBL0]
  Bus Selector1/1 -> [Ib], Ib/1  "<Ib>"
  Mux/1 -> Switch/1
  Switch/1 -> Demux/1
  [SttCBL0] -> Switch1/1
  [SttCBL1] -> Switch1/3
  fail/1 -> Compare To Constant1/1
  Compare To Constant1/1 -> Switch1/2, Switch/2
  Constant/1 -> Cable LR/3(Ib0)

== system MBDMotorSystemUpd1MaxIaLmt/Power Source/Power Source Cs ==
  note: フェール時信号切替
  Vb0 : Inport
  I Load : Inport  Port=2
  fail : Inport  Port=3
  Bus Creator : BusCreator  Inputs=2
  Bus Selector : BusSelector  OutputSignals=Vdc,Ib
  Cs No ESL : Subsystem  mask{CsU=CsU, IsEnableESR=Off, ESRm=ESRm, IsEnableIR=Off, IRM=IRM}
      mask prompts: CsU "コンデンサ容量 [uF]"; IsEnableESR "ESR考慮"; ESRm "ESR [mΩ]"; IsEnableIR "IR考慮"; IRM "IR [MΩ]"
      mask init:
      | Cs  = CsU  * 1.0e-6;
      |     ESR = ESRm * 1.0e-3;
      |     IR  = IRM  * 1.0e6;
      mask TypeOptions IsEnableESR: IsESR/LabelModeActiveChoice | IsESRini/LabelModeActiveChoice
      mask TypeOptions IsEnableIR: isIR/LabelModeActiveChoice
      mask DialogControl ParameterGroupVar Prompt: パラメーター
      mask Display:
      | ss = 'Cs No ESL.';
      | if strcmpi(get_param(gcbh, "IsEnableESR"), 'On')
      |     ss = sprintf('%s\nESR', ss);
      | end
      | if strcmpi(get_param(gcbh, "IsEnableIR"), 'On')
      |     if contains(ss, 'ESR', 'IgnoreCase',true)
      |         ss = sprintf('%s / IR', ss);
      |     else
      |         ss = sprintf('%s\nIR', ss);
      |     end
      | end
      | % cv = evalin("caller","Cs")*1e6;
      | % ss =sprintf('%s\n %g[uF]', ss, cv);
      | ss =sprintf('%s\n %s[uF]', ss, get_param(gcbh, "CsU"));
      | 
      | if strcmpi(get_param(gcbh, "IsEnableESR"), 'On')
      |     % rv = evalin("caller","ESR")*1e3;
      |     % ss = sprintf('%s\n%g[mΩ]', ss, rv);
      |     ss =sprintf('%s\n %s[mΩ]', ss, get_param(gcbh, "ESRm"));
      | end
      | if strcmpi(get_param(gcbh, "IsEnableIR"), 'On')
      |     if contains(ss, 'ESR', 'IgnoreCase',true)
      |         ss = sprintf('%s / ', ss);
      |     else
      |         ss = sprintf('%s\n', ss);
      |     end
      |     % rv = evalin("caller","IR")*1e-6;
      |     % ss = sprintf('%s%g[MΩ]', ss, rv);
      |     ss = sprintf('%s%s[MΩ]', ss, get_param(gcbh, "IRM"));
      | end
      | 
      | disp(ss)
      | % if strcmpi(get_param(gcbh, "IsEnableESR"), 'On')
      | %     ss = sprintf('%s\nESR', ss);
      | % end
      | % if strcmpi(get_param(gcbh, "IsEnableIR"), 'On')
      | %     if contains(ss, 'ESR', 'IgnoreCase',true)
      | %         ss = sprintf('%s / IR', ss);
      | %     else
      | %         ss = sprintf('%s\nIR', ss);
      | %     end
      | % end
  Eb Iout : Subsystem  mask{TypeSource=PS, Cb=Cb, Rb=Rb, IsZinM=Off, Cm=Cm, Rm=Rm, IsZinD=Off, Cd=Cd, Rd=Rd}
      mask prompts: TypeSource "電源ソース"; Cb "キャパシタ容量 [F]"; Rb "内部抵抗 [Ω]"; IsZinM "電荷移動特性考慮"; Cm "容量 [F]"; Rm "抵抗 [Ω]"; IsZinD "拡散特性考慮"; Cd "容量 [F]"; Rd "抵抗 [Ω]"
      mask TypeOptions TypeSource: Source/LabelModeActiveChoice
      mask TypeOptions IsZinM: Zcm/LabelModeActiveChoice
      mask TypeOptions Cm: Zm/Cz
      mask TypeOptions Rm: Zm/Rz
      mask TypeOptions IsZinD: Zcd/LabelModeActiveChoice
      mask TypeOptions Cd: Zd/Cz
      mask TypeOptions Rd: Zd/Rz
      mask DialogControl ParameterGroupVar Prompt: パラメーター
      mask DialogControl Container3 Prompt: 内部インピーダンス
      mask DialogControl Container4 Prompt: 電荷移動特性
      mask DialogControl Container5 Prompt: 拡散特性
      mask Display:
      | ss = get_param(gcbh, "TypeSource");
      | stm = get_param(gcbh, "IsZinM");
      | if strcmpi(stm, 'On')
      |     ss = sprintf('%s\n Zm', ss);
      | end
      | std = get_param(gcbh, "IsZinD");
      | if strcmpi(std, 'On')
      |     if strcmpi(stm, 'On')
      |         ss = sprintf('%s / Zd', ss);
      |     else
      |         ss = sprintf('%s\n Zd', ss);
      |     end
      | end
      | ss = sprintf('%s\n %s[Ω]', ss, get_param(gcbh, "Rb"));
      | if strcmpi(stm, 'On')
      |     ss = sprintf('%s\n %s[F] / %s[Ω]', ss, ...
      |         get_param(gcbh, "Cm"), get_param(gcbh, "Rm"));
      | end
      | if strcmpi(std, 'On')
      |     ss = sprintf('%s\n %s[F] / %s[Ω]', ss, ...
      |         get_param(gcbh, "Cd"), get_param(gcbh, "Rd"));
      | end
      | fprintf('Batt. Iout\n%s', ss)
  Fail Status : MultiPortSwitch  DataPortOrder=Zero-based contiguous  DataPortForDefault=Additional data port  DiagnosticForDefault=Warning  zeroidx=on  SaturateOnIntegerOverflow=off  InputSameDT=off
  Ib0 : Constant  Value=0
  Normal : BusCreator  Inputs=2
  Open : BusCreator  Inputs=2
  Short : BusCreator  Inputs=2
  Vo : Constant  Value=0
  Vdc : Outport
  Ib : Outport  Port=2
  Stt : Outport  Port=3
  wires:
  I Load/1 -> Cs No ESL/1(I Load)
  Cs No ESL/1(Vdc) -> [Vdc]
  Bus Creator/1 -> Stt/1  "PsStt"
  fail/1 -> Fail Status/1
  Eb Iout/1(Ib) -> [Ibb]
  [Vdc] -> Normal/1  "Vdc"
  [Ibb] -> Normal/2  "Ib"
  Normal/1 -> Fail Status/5, Fail Status/2
  Short/1 -> Fail Status/3
  [Vdc] -> Open/1  "Vdc"
  Open/1 -> Fail Status/4
  Vo/1 -> Short/1  "Vdc"
  Fail Status/1 -> Bus Selector/1
  Bus Selector/1 -> [VdcS]  "<Vdc>"
  Bus Selector/2 -> [IbS]  "<Ib>"
  [IbS] -> Cs No ESL/2(Ib)
  [VdcS] -> Vdc/1
  [VdcS] -> Eb Iout/2(V Load)
  Cs No ESL/2(Stt) -> Bus Creator/1
  Eb Iout/3(Stt) -> [VbStt]
  [VbStt] -> Bus Creator/2
  Ib0/1 -> Short/2, Open/2  "Ib"
  [IbS] -> Ib/1
  Vb0/1 -> Eb Iout/1(Vb0)
  Eb Iout/2(Vo) -> Cs No ESL/3(V0in)

== system MBDMotorSystemUpd1MaxIaLmt/Vuvw Input Model/Copper Loss ==
  Idq : Inport
  Ra : Inport  Port=2
  Fcn : Fcn  Expr=u(1)*u(1)+u(2)*u(2)
  Product2 : Product
  Copper loss : Outport
  wires:
  Idq/1 -> Fcn/1
  Fcn/1 -> Product2/1
  Ra/1 -> Product2/2
  Product2/1 -> Copper loss/1

== system MBDMotorSystemUpd1MaxIaLmt/Vuvw Input Model/DQtoUVW1 ==
  dq : Inport
  Pos[deg.] : Inport  Port=2
  Constant : Constant  Value=sqrt(2/3)*[1 -1/2 -1/2; 0 sqrt(3)/2 -sqrt(3)/2]'
  Constant1 : Constant  Value=180
  Degrees to Radians : simulink_extras/Transformations/Degrees to Radians
  Mux1 : Mux  Inputs=2
  Mux2 : Mux  Inputs=2
  Product : Product  Multiplication=Matrix(*)
  Sum : Sum  Inputs=|++
  alpha-phase : Fcn  Expr=u(1)*cos(u(3))-u(2)*sin(u(3))
  beta-phase : Fcn  Expr=u(1)*sin(u(3))+u(2)*cos(u(3))
  UVW : Outport
  wires:
  Mux1/1 -> alpha-phase/1, beta-phase/1
  beta-phase/1 -> Mux2/2  "vBph"
  alpha-phase/1 -> Mux2/1  "vAph"
  Constant/1 -> Product/1
  Product/1 -> UVW/1
  Mux2/1 -> Product/2
  dq/1 -> Mux1/1
  Sum/1 -> Degrees to Radians/1
  Constant1/1 -> Sum/2
  Pos[deg.]/1 -> Sum/1
  Degrees to Radians/1 -> Mux1/2

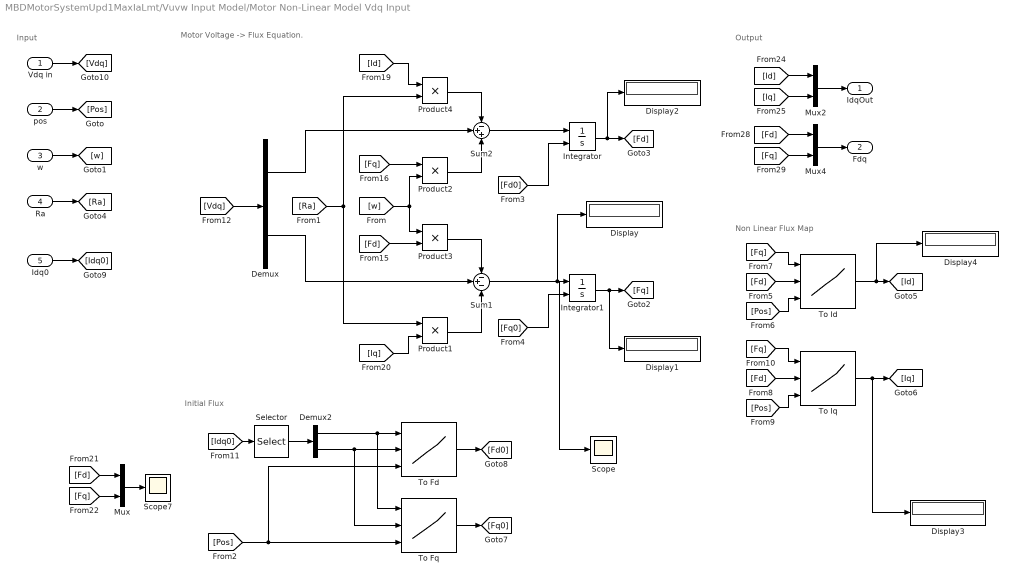
== system MBDMotorSystemUpd1MaxIaLmt/Vuvw Input Model/Motor Non-Linear Model Vdq Input ==
  note: Initial Flux
  note: Input
  note: Output
  note: Motor Voltage -> Flux Equation.
  note: Non Linear Flux Map
  Vdq in : Inport
  pos : Inport  Port=2
  w : Inport  Port=3
  Ra : Inport  Port=4
  Idq0 : Inport  Port=5
  Demux : Demux  Outputs=2
  Demux2 : Demux  Outputs=2
  Display{,1..4} (5 alike) : Display
  Integrator : Integrator  InitialConditionSource=external  ZeroCross=off
  Integrator1 : Integrator  InitialConditionSource=external
  Mux : Mux  Inputs=2
  Mux2 : Mux  Inputs=2
  Mux4 : Mux  Inputs=2
  Product{1..4} (4 alike) : Product
  Scope : Scope
  Scope7 : Scope
  Selector : Selector  InputPortWidth=2  IndexOptions=Index vector (dialog)  Indices=[2 1]  OutputSizes=1
  Sum1 : Sum  Inputs=-+-
  Sum2 : Sum  Inputs=-++
  To Fd : Lookup_n-D  NumberOfTableDimensions=3  BreakpointsForDimension1=xIq  BreakpointsForDimension2=yId  BreakpointsForDimension3=fzTh  BeginIndexSearchUsingPreviousIndexResult=on  Table=fMapD  InternalRulePriority=Speed  RndMeth=Simplest
      settings: InputPortMap=u0,u1,u2
  To Fq : Lookup_n-D  NumberOfTableDimensions=3  BreakpointsForDimension1=xIq  BreakpointsForDimension2=yId  BreakpointsForDimension3=fzTh  BeginIndexSearchUsingPreviousIndexResult=on  Table=fMapQ  InternalRulePriority=Speed  RndMeth=Simplest
      settings: InputPortMap=u0,u1,u2
  To Id : Lookup_n-D  NumberOfTableDimensions=3  BreakpointsForDimension1=xFq  BreakpointsForDimension2=yFd  BreakpointsForDimension3=zTh  BeginIndexSearchUsingPreviousIndexResult=on  Table=iMapD  ExtrapMethod=Clip  InternalRulePriority=Speed  RndMeth=Simplest
      settings: InputPortMap=u0,u1,u2
  To Iq : Lookup_n-D  NumberOfTableDimensions=3  BreakpointsForDimension1=xFq  BreakpointsForDimension2=yFd  BreakpointsForDimension3=zTh  BeginIndexSearchUsingPreviousIndexResult=on  Table=iMapQ  ExtrapMethod=Clip  InternalRulePriority=Speed  RndMeth=Simplest
      settings: InputPortMap=u0,u1,u2
  IdqOut : Outport
  Fdq : Outport  Port=2
  wires:
  Integrator1/1 -> Display1/1, [Fq]
  [Fq] -> To Id/1
  To Id/1 -> Display4/1, [Id]
  [Pos] -> To Id/3
  [Fd] -> To Id/2
  [Pos] -> To Iq/3
  [Fd] -> To Iq/2
  [Fq] -> To Iq/1
  Integrator/1 -> Display2/1, [Fd]
  [Id] -> Product4/1
  Product3/1 -> Sum1/1
  Sum2/1 -> Integrator/1
  Product1/1 -> Sum1/3
  [w] -> Product2/2, Product3/1
  [Fq] -> Product2/1
  [Fd] -> Product3/2
  Sum1/1 -> Display/1, Scope/1, Integrator1/1
  [Iq] -> Product1/2
  Product2/1 -> Sum2/3
  Product4/1 -> Sum2/1
  [Fq] -> Mux/2
  [Fd] -> Mux/1
  To Iq/1 -> Display3/1, [Iq]
  Mux/1 -> Scope7/1
  Demux/1 -> Sum2/2
  Demux/2 -> Sum1/2
  pos/1 -> [Pos]
  Mux2/1 -> IdqOut/1
  [Id] -> Mux2/1
  [Iq] -> Mux2/2
  Mux4/1 -> Fdq/1
  [Fd] -> Mux4/1
  [Fq] -> Mux4/2
  [Ra] -> Product1/1, Product4/2
  w/1 -> [w]
  Ra/1 -> [Ra]
  [Fd0] -> Integrator/2
  [Fq0] -> Integrator1/2
  To Fd/1 -> [Fd0]
  To Fq/1 -> [Fq0]
  Demux2/2 -> To Fq/2, To Fd/2
  [Pos] -> To Fd/3, To Fq/3
  Selector/1 -> Demux2/1
  [Idq0] -> Selector/1
  Demux2/1 -> To Fd/1, To Fq/1
  Idq0/1 -> [Idq0]
  Vdq in/1 -> [Vdq]
  [Vdq] -> Demux/1

== system MBDMotorSystemUpd1MaxIaLmt/Vuvw Input Model/Output Torque  ==
  Idq [A] : Inport
  Fdq [Wb] : Inport  Port=2
  Pos[deg.] : Inport  Port=3
  Demux : Demux  Outputs=2
  Demux1 : Demux  Outputs=2
  Demux2 : Demux  Outputs=2
  Gain1 : Gain  Gain=nPole
  Gain2 : Gain  Gain=1/2
  Product : Product
  Product1 : Product
  Selector : Selector  InputPortWidth=2  IndexOptions=Index vector (dialog)  Indices=[2 1]  OutputSizes=1
  Sum : Sum  Inputs=+|-
  Trq Ripple : Lookup_n-D  NumberOfTableDimensions=3  BreakpointsForDimension1=xIqT  BreakpointsForDimension2=yIdT  BreakpointsForDimension3=zThT  BeginIndexSearchUsingPreviousIndexResult=on  Table=tMap  InternalRulePriority=Speed  RndMeth=Simplest
      settings: InputPortMap=u0,u1,u2
  Trq [Nm] : Outport
  TrqCal [Nm] : Outport  Port=2
  wires:
  Sum/1 -> Gain1/1
  Idq [A]/1 -> Selector/1, Demux1/1
  Gain1/1 -> Gain2/1
  Demux1/2 -> Product/1
  Demux/1 -> Product/2
  Demux/2 -> Product1/2
  Demux1/1 -> Product1/1
  Product/1 -> Sum/1
  Product1/1 -> Sum/2
  Gain2/1 -> TrqCal [Nm]/1
  Pos[deg.]/1 -> Trq Ripple/3
  Trq Ripple/1 -> Trq [Nm]/1
  Demux2/2 -> Trq Ripple/2
  Demux2/1 -> Trq Ripple/1
  Selector/1 -> Demux2/1
  Fdq [Wb]/1 -> Demux/1

== system MBDMotorSystemUpd1MaxIaLmt/Vuvw Input Model/SpdToPos ==
  Spd [rpm] : Inport
  Ini. Pos. Mech. [deg.] : Inport  Port=2
  Demux : Demux  Outputs=3
  Gain : Gain  Gain=360
  Gain2 : Gain  Gain=2*pi
  Gain4 : Gain  Gain=1/60
  Integrator : Integrator  InitialConditionSource=external  InitialCondition=Pos0  WrapState=on  WrappedStateUpperValue=360  WrappedStateLowerValue=0
  Integrator1 : Integrator  InitialConditionSource=external  InitialCondition=Pos0  WrapState=on  WrappedStateUpperValue=360  WrappedStateLowerValue=0
  Mux : Mux  Inputs=3
  Pole : Gain  Gain=Pn
  pos Elec. [deg.] : Outport
  pos. Mech. [deg.] : Outport  Port=2
  w [rad./s] : Outport  Port=3
  wires:
  Demux/3 -> Integrator1/2
  Gain2/1 -> Mux/1
  Gain4/1 -> Gain2/1, Gain/1
  Pole/1 -> Demux/1
  Ini. Pos. Mech. [deg.]/1 -> Mux/3, Integrator/2
  Mux/1 -> Pole/1
  Gain/1 -> Mux/2, Integrator/1
  Demux/2 -> Integrator1/1
  Integrator1/1 -> pos Elec. [deg.]/1
  Integrator/1 -> pos. Mech. [deg.]/1
  Demux/1 -> w [rad./s]/1
  Spd [rpm]/1 -> Gain4/1

== system MBDMotorSystemUpd1MaxIaLmt/Vuvw Input Model/Temp Coefficient1 ==
  Temp : Inport
  BateTemp : Constant  Value=T0
  Coefficient : Gain  Gain=Kt
  Constant : Constant
  Sum : Sum  Inputs=|+-
  Sum1 : Sum  Inputs=|++
  kVal : Outport
  wires:
  Sum1/1 -> kVal/1
  Coefficient/1 -> Sum1/2
  Constant/1 -> Sum1/1
  BateTemp/1 -> Sum/2
  Temp/1 -> Sum/1
  Sum/1 -> Coefficient/1

== system MBDMotorSystemUpd1MaxIaLmt/Vuvw Input Model/UVWtoDQ ==
  UVW : Inport
  Pos[deg.] : Inport  Port=2
  Constant : Constant  Value=sqrt(2/3)*[1 -1/2 -1/2; 0 sqrt(3)/2 -sqrt(3)/2]
  Constant1 : Constant  Value=180
  Degrees to Radians : simulink_extras/Transformations/Degrees to Radians
  Mux1 : Mux  Inputs=2
  Mux2 : Mux  Inputs=2
  Product : Product  Multiplication=Matrix(*)
  Sum : Sum  Inputs=|++
  d-Axis : Fcn  Expr=u(1)*cos(u(3))+u(2)*sin(u(3))
  q-Axis : Fcn  Expr=-u(1)*sin(u(3))+u(2)*cos(u(3))
  dq : Outport
  wires:
  Mux2/1 -> dq/1
  Mux1/1 -> d-Axis/1, q-Axis/1
  q-Axis/1 -> Mux2/2  "vQax"
  d-Axis/1 -> Mux2/1  "vDax"
  UVW/1 -> Product/2
  Constant/1 -> Product/1
  Product/1 -> Mux1/1
  Degrees to Radians/1 -> Mux1/2
  Pos[deg.]/1 -> Sum/1
  Sum/1 -> Degrees to Radians/1
  Constant1/1 -> Sum/2

== system MBDMotorSystemUpd1MaxIaLmt/PM Controller/CalcFreq/LPF ==
  In : Inport  SampleTime=Ts
  Init : Inport  Port=2  SampleTime=Ts
  Constant : Constant  Value=Ts
  Constant1 : Constant  Value=tau
  Delay : Delay  DelayLength=1  InitialConditionSource=Input port
      settings: InputPortMap=u0,p4
  Divide1 : Product  Inputs=*/
  Divide3 : Product  Inputs=*/
  Product : Product
  Product1 : Product
  Sum1 : Sum
  Sum2 : Sum
  Sum3 : Sum  Inputs=-+
  Out : Outport
  wires:
  Constant1/1 -> Divide1/1, Sum1/2
  Constant/1 -> Sum1/1, Divide3/1
  Sum1/1 -> Divide1/2, Divide3/2
  Divide3/1 -> [kX]
  Divide1/1 -> [kY]
  In/1 -> Product/1
  [kX] -> Product/2
  Product/1 -> Sum3/1, Sum2/1
  Sum2/1 -> Out/1, Product1/1
  [kY] -> Product1/2
  Product1/1 -> Delay/1
  Delay/1 -> Sum2/2
  Init/1 -> Sum3/2
  Sum3/1 -> Delay/2

== system MBDMotorSystemUpd1MaxIaLmt/PM Controller/IPM Trq To Id-Iq Request/Torque Rate Limitter ==
  In : Inport
  Time : Inport  Port=2
  Constant : Constant  Value=DltLmt
  Gain : Gain  Gain=-1
  Product : Product
  Saturation Dynamic : simulink/Discontinuities/Saturation Dynamic  OutMin=[]  OutMax=[]  OutDataTypeStr=Inherit: Same as second input  OutDataType=fixdt(1, 16)  OutScaling=2^-10  DoSatur=off
  Sum : Sum  Inputs=|-+
  Sum1 : Sum  Inputs=-+|
  Sum2 : Sum  Inputs=++|
  Unit Delay : UnitDelay  SampleTime=-1  HasFrameUpgradeWarning=on
  Unit Delay1 : UnitDelay  SampleTime=-1  HasFrameUpgradeWarning=on
  Rate Limited : Outport  PortDimensions=1
  wires:
  Saturation Dynamic/1 -> Sum2/2
  Sum/1 -> Product/2
  Unit Delay1/1 -> Sum2/1, Sum1/1
  Constant/1 -> Product/1
  Time/1 -> Unit Delay/1, Sum/2
  Sum1/1 -> Saturation Dynamic/2
  Gain/1 -> Saturation Dynamic/3
  Unit Delay/1 -> Sum/1
  Sum2/1 -> Unit Delay1/1, Rate Limited/1
  In/1 -> Sum1/2
  Product/1 -> Saturation Dynamic/1, Gain/1

== system MBDMotorSystemUpd1MaxIaLmt/PM Controller/Modulator/DQ to UVW ==
  dq : Inport
  Th : Inport  Port=2
  Constant : Constant  Value=sqrt(2/3)*[1 -1/2 -1/2; 0 sqrt(3)/2 -sqrt(3)/2]'
  Constant1 : Constant  Value=180
  Degrees to Radians : simulink_extras/Transformations/Degrees to Radians
  Mux1 : Mux  Inputs=2
  Mux2 : Mux  Inputs=2
  Product : Product  Multiplication=Matrix(*)
  Sum : Sum  Inputs=|++
  alpha-phase : Fcn  Expr=u(1)*cos(u(3))-u(2)*sin(u(3))
  bet-phase : Fcn  Expr=u(1)*sin(u(3))+u(2)*cos(u(3))
  UVW : Outport
  wires:
  Mux2/1 -> Product/2
  Degrees to Radians/1 -> Mux1/2
  alpha-phase/1 -> Mux2/1  "vAph"
  Sum/1 -> Degrees to Radians/1
  bet-phase/1 -> Mux2/2  "vBph"
  Constant1/1 -> Sum/2
  Constant/1 -> Product/1
  Mux1/1 -> alpha-phase/1, bet-phase/1
  Product/1 -> UVW/1
  dq/1 -> Mux1/1
  Th/1 -> Sum/1

== system MBDMotorSystemUpd1MaxIaLmt/PM Controller/Modulator/Over Modulation ==
  Is OvrMod : Inport
  PWM Mode : Inport  Port=2
  Mr : Inport  Port=3
  Merge : Merge
  Ovr. Mod. : Subsystem  TreatAsAtomicUnit=on
  Ovr. Mod. Enable : If
  Through : Subsystem  TreatAsAtomicUnit=on
  Mr* : Outport
  wires:
  Is OvrMod/1 -> Ovr. Mod. Enable/1
  Ovr. Mod. Enable/1 -> Ovr. Mod./Action
  Ovr. Mod. Enable/2 -> Through/Action
  Through/1(Mr*) -> Merge/2
  Ovr. Mod./1(Mr*) -> Merge/1
  Merge/1 -> Mr*/1
  Mr/1 -> Through/1(Mr), Ovr. Mod./2(Mr)
  PWM Mode/1 -> Ovr. Mod./1(PWM Mode)

== system MBDMotorSystemUpd1MaxIaLmt/PM Controller/Modulator/Vz Correction ==
  PWM Mode : Inport
  VaReq : Inport  Port=2
  MaxVa : Inport  Port=3
  DPWM : Subsystem  TreatAsAtomicUnit=on
  Merge : Merge  Inputs=3
  Nothing : Subsystem  TreatAsAtomicUnit=on
  SVM : Subsystem  TreatAsAtomicUnit=on
  Switch Case : SwitchCase  CaseConditions={0, 1}
  Vz : Outport
  wires:
  PWM Mode/1 -> Switch Case/1
  Switch Case/3 -> Nothing/Action
  VaReq/1 -> DPWM/1(VaReq), SVM/1(VaReq)
  SVM/1(Vz) -> Merge/1
  DPWM/1(Vz) -> Merge/2
  Nothing/1(Vz) -> Merge/3
  Switch Case/1 -> SVM/Action
  Switch Case/2 -> DPWM/Action
  Merge/1 -> Vz/1
  MaxVa/1 -> DPWM/2(MaxVa)

== system MBDMotorSystemUpd1MaxIaLmt/PM Controller/PM Feedback Controller/DQ to UVW ==
  dq : Inport
  Th. [deg.] : Inport  Port=2
  Constant : Constant  Value=sqrt(2/3)*[1 -1/2 -1/2; 0 sqrt(3)/2 -sqrt(3)/2]'
  Constant1 : Constant  Value=180
  Degrees to Radians : simulink_extras/Transformations/Degrees to Radians
  Mux1 : Mux  Inputs=2
  Mux2 : Mux  Inputs=2
  Product : Product  Multiplication=Matrix(*)
  Sum : Sum  Inputs=|++
  alpha-phase : Fcn  Expr=u(1)*cos(u(3))-u(2)*sin(u(3))
  beta-phase : Fcn  Expr=u(1)*sin(u(3))+u(2)*cos(u(3))
  UVW : Outport
  wires:
  beta-phase/1 -> Mux2/2  "vBph"
  Constant1/1 -> Sum/2
  Degrees to Radians/1 -> Mux1/2
  alpha-phase/1 -> Mux2/1  "vAph"
  Constant/1 -> Product/1
  Mux2/1 -> Product/2
  Mux1/1 -> beta-phase/1, alpha-phase/1
  Sum/1 -> Degrees to Radians/1
  dq/1 -> Mux1/1
  Th. [deg.]/1 -> Sum/1
  Product/1 -> UVW/1

== system MBDMotorSystemUpd1MaxIaLmt/PM Controller/PM Feedback Controller/UVW to DQ ==
  UVW : Inport
  Th(deg.) : Inport  Port=2
  Constant : Constant  Value=sqrt(2/3)*[1 -1/2 -1/2; 0 sqrt(3)/2 -sqrt(3)/2]
  Constant1 : Constant  Value=180
  Degrees to Radians : simulink_extras/Transformations/Degrees to Radians
  Mux1 : Mux  Inputs=2
  Mux2 : Mux  Inputs=2
  Product : Product  Multiplication=Matrix(*)
  Sum : Sum  Inputs=|++
  d-Axis : Fcn  Expr=u(1)*cos(u(3))+u(2)*sin(u(3))
  q-Axis : Fcn  Expr=-u(1)*sin(u(3))+u(2)*cos(u(3))
  dq : Outport
  wires:
  Product/1 -> Mux1/1
  UVW/1 -> Product/2
  Degrees to Radians/1 -> Mux1/2
  Constant/1 -> Product/1
  Mux2/1 -> dq/1
  Mux1/1 -> d-Axis/1, q-Axis/1
  q-Axis/1 -> Mux2/2  "vQax"
  d-Axis/1 -> Mux2/1  "vDax"
  Th(deg.)/1 -> Sum/1
  Sum/1 -> Degrees to Radians/1
  Constant1/1 -> Sum/2

== system MBDMotorSystemUpd1MaxIaLmt/PM Controller/PM Feedback Controller/dq-Aixs Current Feedback NonLiner Controller ==
  note: FeedBack
  note: Cut off Gain
  Ref : Inport
  Tgt : Inport  Port=2
  P Gain : Inport  Port=3
  I-Gain : Inport  Port=4
  Anti Wup : Inport  Port=5
  Is Vsat : Inport  Port=6  PortDimensions=1
  Cut-off Gain MTPA : Constant  Value=KcT
  Cut-off Gain MTPA1 : Constant  Value=KcW
  Delay : Delay  DelayLength=1
  Discrete-Time Integrator : DiscreteIntegrator  InitialConditionSource=external  SampleTime=-1  ICPrevOutput=DiscIntNeverNeededParam  ICPrevScaledInput=DiscIntNeverNeededParam
  Divide : Product  Inputs=*/
  Product{,1..3} (4 alike) : Product
  Sum : Sum  Inputs=|+-
  Sum1 : Sum  Inputs=+|+
  Sum3 : Sum  Inputs=+-|
  Switch3 : Switch  Criteria=u2 > Threshold  SaturateOnIntegerOverflow=off  InputSameDT=off
  FbVal : Outport
  wires:
  [Kc] -> Product/2
  [Tgt] -> Product3/2
  [KiDQ] -> Product3/1
  Product3/1 -> Discrete-Time Integrator/2
  [KiDQ] -> Product2/1
  Sum3/1 -> Product2/2
  [KpDQ] -> Product1/1
  I-Gain/1 -> [KiDQ]
  P Gain/1 -> [KpDQ]
  Product/1 -> Sum3/1, Product1/2
  Ref/1 -> Sum/1
  Tgt/1 -> Sum/2, [Tgt]
  Product2/1 -> Discrete-Time Integrator/1
  Product1/1 -> Sum1/1
  Discrete-Time Integrator/1 -> Sum1/2
  [KpDQ] -> Divide/2
  Sum1/1 -> FbVal/1
  Anti Wup/1 -> Divide/1
  Sum/1 -> [Err]
  [Err] -> Product/1
  Cut-off Gain MTPA/1 -> Switch3/1
  Cut-off Gain MTPA1/1 -> Switch3/3
  Switch3/1 -> Delay/1
  Is Vsat/1 -> [FlgVfw]
  [FlgVfw] -> Switch3/2
  Divide/1 -> [vAwp]
  [vAwp] -> Sum3/2
  Delay/1 -> [Kc]
